simulink model "kalman_simulink"  (R2021a)
settings: Solver=VariableStepAuto  StartTime=0.0  StopTime=10.0  RelTol=1e-3  EnableMultiTasking=on
libraries: simulink x2
settings Model: Creator=Administrator  LastModifiedBy=86158
settings SolverCC: AlgebraicLoopSolver=TrustRegion
settings DataIOCC: LimitDataPoints=on  ReturnWorkspaceOutputs=off
settings OptimizationCC: LifeSpan=inf
settings DebuggingCC: AllowSymbolicDim=off  SFUnexpectedBacktrackingDiag=warning  SFNoUnconditionalDefaultTransitionDiag=warning  SFExecutionAtInitializationDiag=none  SFMachineParentedDataDiag=warning  ArithmeticOperatorsInVariantConditions=warning
settings ModelReferenceCC: PropagateSignalLabelsOutOfModel=off
settings SFSimCC: SimUseLocalCustomCode=off  CustomCodeUndefinedFunction=UseInterfaceOnly
settings RTWCC: RTWUseLocalCustomCode=off
settings CodeAppCC: StateflowObjectComments=on
settings GRTTargetCC: TargetLangStandard=C89/C90 (ANSI)
settings ConfigComp: CovMetricSettings=dw  CovSaveCumulativeToWorkspaceVar=on  CovSaveSingleToWorkspaceVar=on  CovExternalEMLEnable=off

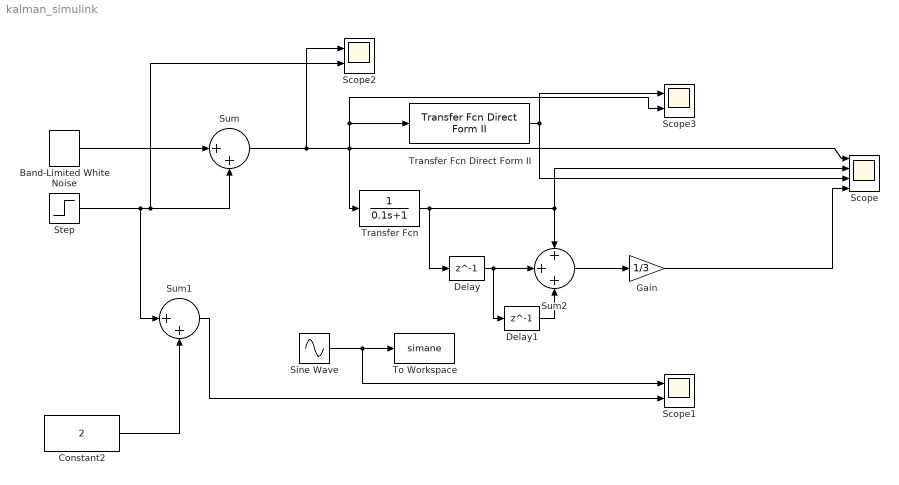
== system kalman_simulink ==
  Band-Limited White Noise : simulink/Sources/Band-Limited White Noise  Cov=[0.04]  Ts=0.1  seed=[23341]
  Constant2 : Constant  Value=2
  Delay : Delay  DelayLength=1  InitialCondition=0  SampleTime=0.05
  Delay1 : Delay  DelayLength=1  InitialCondition=0  SampleTime=0.05
  Gain : Gain  Gain=1/3
  Scope : Scope  NumInputPorts=4
  Scope1 : Scope  NumInputPorts=2
  Scope2 : Scope  NumInputPorts=2
  Scope3 : Scope  NumInputPorts=2
  Sine Wave : Sin  Amplitude=10  Frequency=2  SampleTime=0
  Step : Step  SampleTime=0
  Sum : Sum  Inputs=|++  RndMeth=Simplest  LockScale=on
  Sum1 : Sum  Inputs=|++
  Sum2 : Sum  Inputs=+++  LockScale=on
  To Workspace : ToWorkspace  VariableName=simane  SaveFormat=Timeseries  SampleTime=0.1
  Transfer Fcn : TransferFcn  Denominator=[0.1 1]
  Transfer Fcn Direct Form II : simulink/Additional Math & Discrete/Additional Discrete/Transfer Fcn Direct Form II  NumCoefVec=[1 -1.7 0.72]  DenCoefVec=[0 0]  vinit=0.0  DoSatur=off
      settings: SourceProductBaseCode=SL
  wires:
  Step/1 -> Sum1/1, Scope2/2, Sum/2
  Sum/1 -> Scope2/1, Transfer Fcn/1, Scope/1, Transfer Fcn Direct Form II/1, Scope3/2
  Sine Wave/1 -> Scope1/1, To Workspace/1
  Constant2/1 -> Sum1/2
  Sum1/1 -> Scope1/2
  Transfer Fcn Direct Form II/1 -> Scope3/1, Scope/3
  Transfer Fcn/1 -> Sum2/1, Scope/2, Delay/1
  Delay/1 -> Delay1/1, Sum2/2
  Sum2/1 -> Gain/1
  Delay1/1 -> Sum2/3
  Gain/1 -> Scope/4
  Band-Limited White Noise/1 -> Sum/1
